simulink model "car_sim"  (R2023a)
settings: Solver=FixedStepAuto  StartTime=0.0  StopTime=20  FixedStep=.01  RelTol=1e-3
values from neighbouring files (symbols this model uses):
  cg = 13/12    (= 1.08333333333)    [car_script.m]    (also in car_script_FY_lookup.m; car_script_Pacejka4.m)
  chassis_k = 1000    [car_script.m]    (also in car_script_FY_lookup.m; car_script_Pacejka4.m)
  dist = zeros(1, length(road_height_right))    [car_script_FY_lookup.m]    (also in car_script_Pacejka4.m)
  f_anti = .2    (= 0.2)    [car_script.m]    (also in car_script_FY_lookup.m; car_script_Pacejka4.m)
  f_arb = 202.9*12    (= 2434.8)    [car_script.m]    (also in car_script_FY_lookup.m; car_script_Pacejka4.m)
  f_c = f_damp_ratio*(2*sqrt(f_sprung*f_spring/(32.17*2)))    [car_script.m]    (also in car_script_FY_lookup.m; car_script_Pacejka4.m)
  f_MR_arb = .4    (= 0.4)    [car_script.m]    (also in car_script_FY_lookup.m; car_script_Pacejka4.m)
  f_MR_spring = .99    (= 0.99)    [car_script.m]    (also in car_script_FY_lookup.m; car_script_Pacejka4.m)
  f_rc = 1/12    (= 0.0833333333333)    [car_script.m]    (also in car_script_FY_lookup.m; car_script_Pacejka4.m)
  f_spring = 250*12    (= 3000)    [car_script.m]    (also in car_script_FY_lookup.m; car_script_Pacejka4.m)
  f_sprung = total_weight*weight_distribution-f_unsprung    (= 276.76)    [car_script.m]    (also in car_script_FY_lookup.m; car_script_Pacejka4.m)
  f_unsprung = 48.24    [car_script.m]    (also in car_script_FY_lookup.m; car_script_Pacejka4.m)
  f_unsprung_cg = 6/12    (= 0.5)    [car_script.m]    (also in car_script_FY_lookup.m; car_script_Pacejka4.m)
  fy_slip_angle_lookup = [fy_slip_angle_lookup, -flip(fy_slip_angle_lookup(:,1:15),2)]    [car_script.m]    (also in car_script_FY_lookup.m)
  Izz = 500    [car_script.m]    (also in car_script_FY_lookup.m; car_script_Pacejka4.m)
  r_anti = .2    (= 0.2)    [car_script.m]    (also in car_script_FY_lookup.m; car_script_Pacejka4.m)
  r_arb = 108.66*12    (= 1303.92)    [car_script.m]    (also in car_script_FY_lookup.m; car_script_Pacejka4.m)
  r_c = r_damp_ratio*(2*sqrt(r_sprung*r_spring/(32.17*2)))    [car_script.m]    (also in car_script_FY_lookup.m; car_script_Pacejka4.m)
  r_MR_arb = .25    (= 0.25)    [car_script.m]    (also in car_script_FY_lookup.m; car_script_Pacejka4.m)
  r_MR_spring = .96    (= 0.96)    [car_script.m]    (also in car_script_FY_lookup.m; car_script_Pacejka4.m)
  r_rc = 2/12    (= 0.166666666667)    [car_script.m]    (also in car_script_FY_lookup.m; car_script_Pacejka4.m)
  r_spring = 150*12    (= 1800)    [car_script.m]    (also in car_script_FY_lookup.m; car_script_Pacejka4.m)
  r_sprung = total_weight*weight_distribution-r_unsprung    (= 277.44)    [car_script.m]    (also in car_script_FY_lookup.m; car_script_Pacejka4.m)
  r_unsprung = 47.56    [car_script.m]    (also in car_script_FY_lookup.m; car_script_Pacejka4.m)
  r_unsprung_cg = 6/12    (= 0.5)    [car_script.m]    (also in car_script_FY_lookup.m; car_script_Pacejka4.m)
  road_height_left = [zeros(1,10000)]    [car_script.m]    (also in car_script_FY_lookup.m; car_script_Pacejka4.m)
  road_height_right = [zeros(1,10000)]    [car_script.m]    (also in car_script_FY_lookup.m; car_script_Pacejka4.m)
  timestep = .01    (= 0.01)    [car_script.m]    (also in car_script_FY_lookup.m; car_script_Pacejka4.m)
  tire_c = .1*(2*sqrt(tire_k*f_unsprung/(2*32.17)))    [car_script.m]    (also in car_script_FY_lookup.m; car_script_Pacejka4.m)
  tire_k = 989*12    (= 11868)    [car_script.m]    (also in car_script_FY_lookup.m; car_script_Pacejka4.m)
  total_unsprung = f_unsprung + r_unsprung    (= 95.8)    [car_script.m]    (also in car_script_FY_lookup.m; car_script_Pacejka4.m)
  total_weight = 650    [car_script.m]    (also in car_script_FY_lookup.m; car_script_Pacejka4.m)
  track = 48/12    (= 4)    [car_script.m]    (also in car_script_FY_lookup.m; car_script_Pacejka4.m)
  vx_o = 51.3333    [car_script.m]    (also in car_script_FY_lookup.m; car_script_Pacejka4.m = 51.33)
  wheelbase = 60.5/12    (= 5.04166666667)    [car_script.m]    (also in car_script_FY_lookup.m; car_script_Pacejka4.m)
libraries: simulink_extras x1, simulink x1
(part 2 of 2)

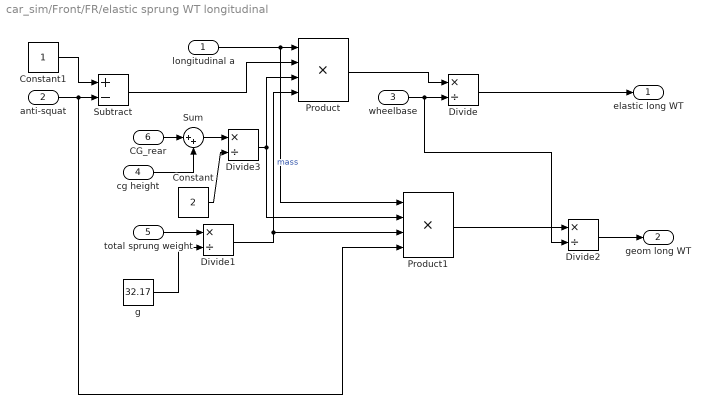
== system car_sim/Front/FR/elastic sprung WT longitudinal ==
  longitudinal a : Inport
  anti-squat : Inport  Port=2
  wheelbase : Inport  Port=3
  cg height : Inport  Port=4
  total sprung weight : Inport  Port=5
  CG_rear : Inport  Port=6
  Constant : Constant  Value=2
  Constant1 : Constant
  Divide{,1..3} (4 alike) : Product  Inputs=*/
  Product : Product  Inputs=4
  Product1 : Product  Inputs=4
  Subtract : Sum  Inputs=+-
  Sum : Sum  Inputs=|++
  g : Constant  Value=32.17
  elastic long WT : Outport
  geom long WT : Outport  Port=2
  wires:
  Product/1 -> Divide/1
  longitudinal a/1 -> Product1/1, Product/1
  anti-squat/1 -> Product1/4, Subtract/2
  Constant1/1 -> Subtract/1
  Subtract/1 -> Product/2
  total sprung weight/1 -> Divide1/1
  g/1 -> Divide1/2
  Divide1/1 -> Product/4, Product1/3  "mass"
  wheelbase/1 -> Divide2/2, Divide/2
  Divide2/1 -> geom long WT/1
  Product1/1 -> Divide2/1
  Divide/1 -> elastic long WT/1
  CG_rear/1 -> Sum/1
  cg height/1 -> Sum/2
  Sum/1 -> Divide3/1
  Constant/1 -> Divide3/2
  Divide3/1 -> Product/3, Product1/2

== system car_sim/Front/FR/unsprung WT lateral ==
  front unsprung cg height : Inport
  lateral a : Inport  Port=2
  track : Inport  Port=3
  front unsprung weight : Inport  Port=4
  2*g : Constant  Value=32.17
  Divide : Product  Inputs=*/
  Divide1 : Product  Inputs=*/
  Product : Product  Inputs=3
  lat WT : Outport
  wires:
  Divide/1 -> lat WT/1
  Product/1 -> Divide/1
  lateral a/1 -> Product/1
  front unsprung weight/1 -> Divide1/1
  2*g/1 -> Divide1/2
  Divide1/1 -> Product/2
  front unsprung cg height/1 -> Product/3
  track/1 -> Divide/2

== system car_sim/Rear/RL/ unsprung WT longitudinal ==
  longitudinal a : Inport
  wheelbase : Inport  Port=2
  front unsprung weight cg height : Inport  Port=3
  total unsprung weight : Inport  Port=4
  Constant : Constant  Value=32.17
  Divide : Product  Inputs=*/
  Divide1 : Product  Inputs=*/
  Product : Product  Inputs=3
  long WT : Outport
  wires:
  Divide/1 -> long WT/1
  Product/1 -> Divide/1
  longitudinal a/1 -> Product/1
  front unsprung weight cg height/1 -> Product/3
  total unsprung weight/1 -> Divide1/1
  Constant/1 -> Divide1/2
  Divide1/1 -> Product/2  "mass"
  wheelbase/1 -> Divide/2

== system car_sim/Rear/RL/elastic sprung WT lateral ==
  CG h : Inport
  lateral a : Inport  Port=2
  track : Inport  Port=3
  rear RC : Inport  Port=4
  front sprung weight : Inport  Port=5
  road height : Inport  Port=6
  Divide : Product  Inputs=*/
  Divide1 : Product  Inputs=*/
  Divide2 : Product  Inputs=*/
  Product : Product  Inputs=3
  Product1 : Product  Inputs=3
  Subtract : Sum  Inputs=+-
  Sum : Sum  Inputs=|++
  g : Constant  Value=32.17
  elastic lat WT : Outport
  geom lat WT : Outport  Port=2
  wires:
  Divide/1 -> elastic lat WT/1
  track/1 -> Divide2/2, Divide/2
  Product/1 -> Divide/1
  CG h/1 -> Subtract/1
  Subtract/1 -> Product/3
  lateral a/1 -> Product1/2, Product/1
  rear RC/1 -> Product1/1, Sum/2
  front sprung weight/1 -> Divide1/1
  g/1 -> Divide1/2
  Divide1/1 -> Product1/3, Product/2  "mass"
  Product1/1 -> Divide2/1
  Divide2/1 -> geom lat WT/1
  road height/1 -> Sum/1
  Sum/1 -> Subtract/2

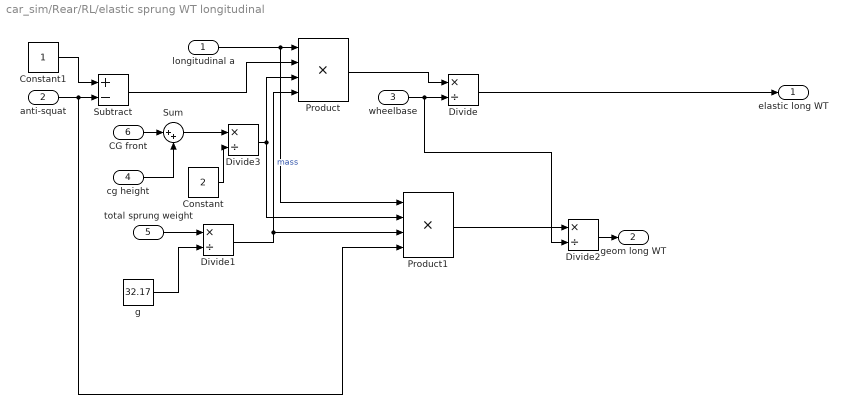
== system car_sim/Rear/RL/elastic sprung WT longitudinal ==
  longitudinal a : Inport
  anti-squat : Inport  Port=2
  wheelbase : Inport  Port=3
  cg height : Inport  Port=4
  total sprung weight : Inport  Port=5
  CG front : Inport  Port=6
  Constant : Constant  Value=2
  Constant1 : Constant
  Divide{,1..3} (4 alike) : Product  Inputs=*/
  Product : Product  Inputs=4
  Product1 : Product  Inputs=4
  Subtract : Sum  Inputs=+-
  Sum : Sum  Inputs=|++
  g : Constant  Value=32.17
  elastic long WT : Outport
  geom long WT : Outport  Port=2
  wires:
  Product/1 -> Divide/1
  longitudinal a/1 -> Product1/1, Product/1
  anti-squat/1 -> Product1/4, Subtract/2
  Constant1/1 -> Subtract/1
  Subtract/1 -> Product/2
  total sprung weight/1 -> Divide1/1
  g/1 -> Divide1/2
  Divide1/1 -> Product/4, Product1/3  "mass"
  wheelbase/1 -> Divide2/2, Divide/2
  Divide2/1 -> geom long WT/1
  Product1/1 -> Divide2/1
  Divide/1 -> elastic long WT/1
  CG front/1 -> Sum/1
  cg height/1 -> Sum/2
  Sum/1 -> Divide3/1
  Constant/1 -> Divide3/2
  Divide3/1 -> Product/3, Product1/2

== system car_sim/Rear/RL/unsprung WT lateral ==
  front unsprung cg height : Inport
  lateral a : Inport  Port=2
  track : Inport  Port=3
  front unsprung weight : Inport  Port=4
  Divide : Product  Inputs=*/
  Divide1 : Product  Inputs=*/
  Product : Product  Inputs=3
  g : Constant  Value=32.17
  lat WT : Outport
  wires:
  Divide/1 -> lat WT/1
  Product/1 -> Divide/1
  lateral a/1 -> Product/1
  front unsprung weight/1 -> Divide1/1
  g/1 -> Divide1/2
  Divide1/1 -> Product/2
  front unsprung cg height/1 -> Product/3
  track/1 -> Divide/2

== system car_sim/Rear/RR/ unsprung WT longitudinal ==
  longitudinal a : Inport
  wheelbase : Inport  Port=2
  front unsprung weight cg height : Inport  Port=3
  total unsprung weight : Inport  Port=4
  Constant : Constant  Value=32.17
  Divide : Product  Inputs=*/
  Divide1 : Product  Inputs=*/
  Product : Product  Inputs=3
  long WT : Outport
  wires:
  Divide/1 -> long WT/1
  Product/1 -> Divide/1
  longitudinal a/1 -> Product/1
  front unsprung weight cg height/1 -> Product/3
  total unsprung weight/1 -> Divide1/1
  Constant/1 -> Divide1/2
  Divide1/1 -> Product/2  "mass"
  wheelbase/1 -> Divide/2

== system car_sim/Rear/RR/elastic sprung WT lateral ==
  CG h : Inport
  lateral a : Inport  Port=2
  track : Inport  Port=3
  rear RC : Inport  Port=4
  front sprung weight : Inport  Port=5
  road height : Inport  Port=6
  Divide : Product  Inputs=*/
  Divide1 : Product  Inputs=*/
  Divide2 : Product  Inputs=*/
  Product : Product  Inputs=3
  Product1 : Product  Inputs=3
  Subtract : Sum  Inputs=+-
  Sum : Sum  Inputs=|++
  g : Constant  Value=32.17
  elastic lat WT : Outport
  geom lat WT : Outport  Port=2
  wires:
  Divide/1 -> elastic lat WT/1
  track/1 -> Divide2/2, Divide/2
  Product/1 -> Divide/1
  CG h/1 -> Subtract/1
  Subtract/1 -> Product/3
  lateral a/1 -> Product1/2, Product/1
  rear RC/1 -> Sum/2, Product1/1
  front sprung weight/1 -> Divide1/1
  g/1 -> Divide1/2
  Divide1/1 -> Product1/3, Product/2  "mass"
  Product1/1 -> Divide2/1
  Divide2/1 -> geom lat WT/1
  road height/1 -> Sum/1
  Sum/1 -> Subtract/2

== system car_sim/Rear/RR/elastic sprung WT longitudinal ==
  longitudinal a : Inport
  anti-squat : Inport  Port=2
  wheelbase : Inport  Port=3
  cg height : Inport  Port=4
  total sprung weight : Inport  Port=5
  CG front : Inport  Port=6
  Constant : Constant  Value=2
  Constant1 : Constant
  Divide{,1..3} (4 alike) : Product  Inputs=*/
  Product : Product  Inputs=4
  Product1 : Product  Inputs=4
  Subtract : Sum  Inputs=+-
  Sum : Sum  Inputs=|++
  g : Constant  Value=32.17
  elastic long WT : Outport
  geom long WT : Outport  Port=2
  wires:
  Product/1 -> Divide/1
  longitudinal a/1 -> Product1/1, Product/1
  anti-squat/1 -> Product1/4, Subtract/2
  Constant1/1 -> Subtract/1
  Subtract/1 -> Product/2
  total sprung weight/1 -> Divide1/1
  g/1 -> Divide1/2
  Divide1/1 -> Product/4, Product1/3  "mass"
  wheelbase/1 -> Divide2/2, Divide/2
  Divide2/1 -> geom long WT/1
  Product1/1 -> Divide2/1
  Divide/1 -> elastic long WT/1
  CG front/1 -> Sum/1
  cg height/1 -> Sum/2
  Constant/1 -> Divide3/2
  Sum/1 -> Divide3/1
  Divide3/1 -> Product1/2, Product/3

== system car_sim/Rear/RR/unsprung WT lateral ==
  front unsprung cg height : Inport
  lateral a : Inport  Port=2
  track : Inport  Port=3
  front unsprung weight : Inport  Port=4
  Divide : Product  Inputs=*/
  Divide1 : Product  Inputs=*/
  Product : Product  Inputs=3
  g : Constant  Value=32.17
  lat WT : Outport
  wires:
  Divide/1 -> lat WT/1
  Product/1 -> Divide/1
  lateral a/1 -> Product/1
  front unsprung weight/1 -> Divide1/1
  g/1 -> Divide1/2
  Divide1/1 -> Product/2
  front unsprung cg height/1 -> Product/3
  track/1 -> Divide/2

== matlab function car_sim/MATLAB Function ==
  data: time input; long_a output
function long_a = fcn(time)

long_a = 0;

== matlab function car_sim/Road surface/MATLAB Function ==
  data: dist_traveled input; FR_surface output size=1; dist input; road_height_right input; road_height_left input; RR_surface output size=1; FL_surface output size=1; RL_surface output size=1; wheelbase input; CG_vel input; FR_vel output size=1; RR_vel output size=1; FL_vel output size=1; RL_vel output size=1
function [FR_surface, RR_surface, FL_surface, RL_surface, FR_vel, RR_vel, FL_vel, RL_vel] = fcn(dist_traveled, dist, road_height_right, road_height_left, wheelbase, CG_vel)

front_wheels_pos = dist_traveled+wheelbase;
i = 0;
while front_wheels_pos/dist(end) > 1
    front_wheels_pos = front_wheels_pos - dist(end);
    i = i + 1;
end

rear_wheels_pos = dist_traveled;
j = 0;
while rear_wheels_pos/dist(end) > 1
    rear_wheels_pos = rear_wheels_pos - dist(end);
    j = j + 1;
end

rear_wheels_pos = round(rear_wheels_pos*10)/10;
col = find(abs(dist-rear_wheels_pos) < .001);

RR_surface_temp = road_height_right(col,1);
RR_surface = RR_surface_temp(1);
RL_surface_temp = road_height_left(col,1);
RL_surface = RL_surface_temp(1);


if col ~= 1
    RR_vel_temp = CG_vel*(road_height_right(col,1)-road_height_right(col-1,1))/(dist(col,1)-dist(col-1,1));
    RR_vel = RR_vel_temp(1);
    RL_vel_temp = CG_vel*(road_height_left(col,1)-road_height_left(col-1,1))/(dist(col,1)-dist(col-1,1));
    RL_vel = RL_vel_temp(1);
else
    RR_vel = 0;
    RL_vel = 0;
end

front_wheels_pos = round(front_wheels_pos*10)/10;
col = find(abs(dist-front_wheels_pos) < .001);

FR_surface_temp = road_height_right(col,1);
FR_surface = FR_surface_temp(1);
FL_surface_temp = road_height_left(col,1);
FL_surface = FL_surface_temp(1);



if col ~= 1
    FR_vel_temp = CG_vel*(road_height_right(col,1)-road_height_right(col-1,1))/(dist(col,1)-dist(col-1,1));
    FR_vel = FR_vel_temp(1);
    FL_vel_temp = CG_vel*(road_height_left(col,1)-road_height_left(col-1,1))/(dist(col,1)-dist(col-1,1));
    FL_vel = FL_vel_temp(1);
else
    FR_vel = 0;
    FL_vel = 0;
end

== matlab function car_sim/Chassis torsion/MATLAB Function ==
  data: sprung_height_FR input; FR output; sprung_height_FL input; sprung_height_RR input; sprung_height_RL input; track input; chassis_torsional_stiffness input; wheelbase input; FL output; RR output; RL output; CG_f output; CG_r output; roll output
function [FR, FL, RR, RL, CG_f, CG_r, roll] = fcn(sprung_height_FR, sprung_height_FL, sprung_height_RR, sprung_height_RL, track, chassis_torsional_stiffness, wheelbase)

sprung_height_FR = floor(sprung_height_FR*100)/100;
sprung_height_FL = floor(sprung_height_FL*100)/100;
sprung_height_RR = floor(sprung_height_RR*100)/100;
sprung_height_RL = floor(sprung_height_RL*100)/100;

f_roll_angle = atan((sprung_height_FL - sprung_height_FR)/track);
r_roll_angle = atan((sprung_height_RL - sprung_height_RR)/track);
roll = (f_roll_angle + r_roll_angle)/2;
left_pitch_angle = atan((sprung_height_RL - sprung_height_FL)/wheelbase);
right_pitch_angle = atan((sprung_height_RR - sprung_height_FR)/wheelbase);

delta_lat = f_roll_angle - r_roll_angle; 
delta_long = left_pitch_angle - right_pitch_angle; 

front_back_couple = chassis_torsional_stiffness*delta_lat/wheelbase;  
left_right_couple = chassis_torsional_stiffness*delta_long/track;  

% positive front back cooresponds to a more rightwards leaning roll in the front
% positive left right cooresponds to more pitch in the left side


FR = front_back_couple;
FL = -front_back_couple;
RR = -FR;
RL = -FL;

if left_right_couple < 0
    FR = FR - left_right_couple;
    RR = RR + left_right_couple;
    FL = FL + left_right_couple;
    RL = RL - left_right_couple;
else
    FR = FR + left_right_couple;
    RR = RR - left_right_couple;
    FL = FL - left_right_couple;
    RL = RL + left_right_couple;
end

CG_f = (sprung_height_FR + sprung_height_FL)/2;
CG_r = (sprung_height_RR + sprung_height_RL)/2;

== matlab function car_sim/traversed angle/MATLAB Function ==
  data: u input; y output
function y = fcn(u)

if u == 0
    y = inf;
else
    y = u;
end

== matlab function car_sim/steering -> lateral acceleration/MATLAB Function1 ==
  data: fr_tire_angle input size=1; fl_tire_angle input; lat_a output size=1; x_v input size=1; y_v input size=1; slip_angle_lookup input; wheelbase input size=1; track input size=1; Fz_fr input size=1; Fz_fl input size=1; Fz_rr input; Fz_rl input; Izz input size=1; yaw_v input size=1; yaw_a output size=1; total_weight input size=1; radius output; yaw_angle input; theta input; lat_v output; long_v output; f_lat_f output; r_lat_f output; yaw_moment output
function [lat_a, yaw_a, radius, lat_v, long_v, f_lat_f, r_lat_f, yaw_moment] = fcn(fr_tire_angle,fl_tire_angle, x_v, y_v, slip_angle_lookup, wheelbase, track, Fz_fr, Fz_fl, Fz_rr, Fz_rl, Izz, yaw_v, total_weight, yaw_angle, theta)

weight_distribution = (Fz_fr+Fz_fl)/(Fz_fr+Fz_fl+Fz_rr+Fz_rl);
tire_model_correction = 1.7/2.4;

% vectors for each wheel w.r.t CG
r_fr = [wheelbase*(1-weight_distribution);-track/2;0];
r_fl = [wheelbase*(1-weight_distribution);track/2;0];
r_rr = [-wheelbase*weight_distribution;-track/2;0];
r_rl = [-wheelbase*weight_distribution; track/2;0];

r_f_mag = sqrt((wheelbase*(1-weight_distribution))^2+(track/2)^2);
r_r_mag = sqrt((wheelbase*weight_distribution)^2+(track/2)^2);

% do the cross product to get the linear velocity components due to yaw velocity
yaw = [0;0;yaw_v];
fr_yaw = cross(r_fr,yaw);
fl_yaw = cross(r_fl,yaw);
rr_yaw = cross(r_rr,yaw);
rl_yaw = cross(r_rl,yaw);

% get the velocity of each wheel
fr_x_v = x_v - fr_yaw(1);
fr_y_v = y_v - fr_yaw(2);

fl_x_v = x_v - fl_yaw(1);
fl_y_v = y_v - fl_yaw(2);

rr_x_v = x_v - rr_yaw(1);
rr_y_v = y_v - rr_yaw(2);

rl_x_v = x_v - rl_yaw(1);
rl_y_v = y_v - rl_yaw(2);

% compute the slip angles of each tire (not counting front wheel toe)
if fr_x_v ~= 0
    fr_CG_v_angle = -tan(fr_y_v/double(fr_x_v));
elseif fr_y_v ~= 0
    fr_CG_v_angle = -sign(fr_y_v)*90;
else
    fr_CG_v_angle = 0;
end 

if fl_x_v ~= 0
    fl_CG_v_angle = -tan(fl_y_v/double(fl_x_v));
elseif fl_y_v ~= 0
    fl_CG_v_angle = -sign(fl_y_v)*90;
else
    fl_CG_v_angle = 0;
end 

if rr_x_v ~= 0
    rr_CG_v_angle = -tan(rr_y_v/double(rr_x_v));
elseif rr_y_v ~= 0 
    rr_CG_v_angle = -sign(rr_y_v)*90;
else
    rr_CG_v_angle = 0;
end

if rl_x_v ~= 0
    rl_CG_v_angle = -tan(rl_y_v/double(rl_x_v));
elseif rr_y_v ~= 0 
    rl_CG_v_angle = -sign(rl_y_v)*90;
else
    rl_CG_v_angle = 0;
end

% final slip angles
fr_slip_angle = double(fr_tire_angle + fr_CG_v_angle);
fl_slip_angle = double(fl_tire_angle + fl_CG_v_angle);
rr_slip_angle = double(rr_CG_v_angle);
rl_slip_angle = double(rl_CG_v_angle);

% get the lateral forces on each tire 
fr_lat_f_temp = slip_angle_to_fy(fr_slip_angle, slip_angle_lookup, -Fz_fr);
fr_lat_f = tire_model_correction*fr_lat_f_temp(1);
fl_lat_f_temp = slip_angle_to_fy(fl_slip_angle, slip_angle_lookup, -Fz_fl);
fl_lat_f = tire_model_correction*fl_lat_f_temp(1);
rr_lat_f_temp = slip_angle_to_fy(rr_slip_angle, slip_angle_lookup, -Fz_rr);
rr_lat_f = tire_model_correction*rr_lat_f_temp(1);
rl_lat_f_temp = slip_angle_to_fy(rl_slip_angle, slip_angle_lookup, -Fz_rl);
rl_lat_f = tire_model_correction*rl_lat_f_temp(1);

% now longitudinal 
fr_long_f = (-Fz_fr)*1.7; % approximate frictional force from tires, which is creating a moment on the CG
fl_long_f = (-Fz_fl)*1.7;
rr_long_f = (-Fz_rr)*1.7;
rl_long_f = (-Fz_rl)*1.7;

% the front forces are all in the tires' frame, so we need to put it in the CG's frame
fr_lat_f_CG = fr_lat_f*cos(fr_tire_angle)+fr_long_f*sin(fr_tire_angle);
fr_long_f_CG = -fr_lat_f*sin(fr_tire_angle)+fr_long_f*cos(fr_tire_angle);
fl_lat_f_CG = fl_lat_f*cos(fl_tire_angle)+fl_long_f*sin(fl_tire_angle);
fl_long_f_CG = -fl_lat_f*sin(fl_tire_angle)+fl_long_f*cos(fl_tire_angle);

f_lat_f = fr_lat_f_CG+fl_lat_f_CG;
r_lat_f = rr_lat_f+rl_lat_f;

lat_a_temp = (f_lat_f+r_lat_f)/(total_weight/32.17);
lat_a = lat_a_temp(1);

radius = (x_v^2+y_v^2)/lat_a;

lat_v =  -sqrt(x_v^2+y_v^2)*sin(yaw_angle-theta);
long_v = sqrt(x_v^2+y_v^2)*cos(yaw_angle-theta);

if abs(theta-yaw_angle) < .006
    scrub_moment_r = 0;
    scrub_moment_fr = 0;
    scrub_moment_fl = 0;
else
    scrub_moment_r = (-Fz_rr*r_r_mag-Fz_rl*r_r_mag)*1.7;
    scrub_moment_fr = (-Fz_fr*r_f_mag)*1.7;
    scrub_moment_fl = (-Fz_fl*r_f_mag)*1.7;
end

moment_fr = cross(r_fr,[fr_long_f_CG;fr_lat_f_CG;0]);
moment_fl = cross(r_fl,[fl_long_f_CG;fl_lat_f_CG;0]);
moment_rr = cross(r_rr,[rr_long_f;rr_lat_f;0]);
moment_rl = cross(r_rl,[rl_long_f;rl_lat_f;0]);

yaw_moment = scrub_moment_r*sign(theta-yaw_angle)+scrub_moment_fr*sign(theta-yaw_angle-fr_tire_angle)+scrub_moment_fl*sign(theta-yaw_angle-fl_tire_angle)+moment_fr(3)+moment_rr(3)+moment_fl(3)+moment_rl(3);

yaw_a_temp = 1/Izz*yaw_moment;
yaw_a = yaw_a_temp(1);

end

function fy = slip_angle_to_fy(slip, slip_angle_lookup, Fz)
    slip_float = rad2deg(double(slip));
    if slip_float == 0
        fy = 0;
        return
    end

    % set a bound on the slip angle (in case)
    if slip_float > 15
        slip_float = 15;
    elseif slip_float < -15
        slip_float = -15;
    end

    % find the upper and lower slip angle
    slip_angles = [-15,-14,-13,-12,-11,-10,-9,-8,-7,-6,-5,-4,-3,-2,-1,0,1,2,3,4,5,6,7,8,9,10,11,12,13,14,15];
    if slip_float > 0
        slip_angle_lower = find(slip_angles(1,:) == floor(slip_float));
        slip_angle_higher = slip_angle_lower + 1;
    else
        slip_angle_lower = find(slip_angles(1,:) == ceil(slip_float));
        slip_angle_higher = slip_angle_lower - 1;
    end
    if slip_angle_higher == 32 % slip angle is 15
        slip_angle_higher = 31; % so we dont end up interpolating
    end
    if slip_angle_lower == 1 % slip angle is -15
        slip_angle_higher = 1; 
    end

    if Fz >= 350 % treat as if Fz is 350, interpolate once
        fy = slip_angle_lookup(5,slip_angle_lower) + (slip_angle_lookup(5,slip_angle_higher)-slip_angle_lookup(5,slip_angle_lower))*abs(slip_float-slip_angles(slip_angle_lower));
    elseif Fz < 50 % interpolate on Fz = 50 and multiply by the fraction Fz/50
        fy = Fz/50*(slip_angle_lookup(1,slip_angle_lower) + (slip_angle_lookup(1,slip_angle_higher)-slip_angle_lookup(1,slip_angle_lower))*abs(slip_float-slip_angles(slip_angle_lower)));
    else % Fz lies in between
        if Fz >= 250
            fy_high = slip_angle_lookup(5,slip_angle_lower) + (slip_angle_lookup(5,slip_angle_higher)-slip_angle_lookup(5,slip_angle_lower))*abs(slip_float-slip_angles(slip_angle_lower));
            fy_low = slip_angle_lookup(4,slip_angle_lower) + (slip_angle_lookup(4,slip_angle_higher)-slip_angle_lookup(4,slip_angle_lower))*abs(slip_float-slip_angles(slip_angle_lower));
            fy = fy_low + (Fz-250)*(fy_high - fy_low)/100;
        elseif Fz >= 150
            fy_high = slip_angle_lookup(4,slip_angle_lower) + (slip_angle_lookup(4,slip_angle_higher)-slip_angle_lookup(4,slip_angle_lower))*abs(slip_float-slip_angles(slip_angle_lower));
            fy_low = slip_angle_lookup(3,slip_angle_lower) + (slip_angle_lookup(3,slip_angle_higher)-slip_angle_lookup(3,slip_angle_lower))*abs(slip_float-slip_angles(slip_angle_lower));
            fy = fy_low + (Fz-150)*(fy_high - fy_low)/100;
        elseif Fz >= 100
            fy_high = slip_angle_lookup(3,slip_angle_lower) + (slip_angle_lookup(3,slip_angle_higher)-slip_angle_lookup(3,slip_angle_lower))*abs(slip_float-slip_angles(slip_angle_lower));
            fy_low = slip_angle_lookup(2,slip_angle_lower) + (slip_angle_lookup(2,slip_angle_higher)-slip_angle_lookup(2,slip_angle_lower))*abs(slip_float-slip_angles(slip_angle_lower));
            fy = fy_low + (Fz-100)*(fy_high - fy_low)/50;
        else
            fy_high = slip_angle_lookup(2,slip_angle_lower) + (slip_angle_lookup(2,slip_angle_higher)-slip_angle_lookup(2,slip_angle_lower))*abs(slip_float-slip_angles(slip_angle_lower));
            fy_low = slip_angle_lookup(1,slip_angle_lower) + (slip_angle_lookup(1,slip_angle_higher)-slip_angle_lookup(1,slip_angle_lower))*abs(slip_float-slip_angles(slip_angle_lower));
            fy = fy_low + (Fz-50)*(fy_high - fy_low)/50;
        end
    end

end
